simulink model "new_inkine_2020"  (R2022b)
settings: Solver=FixedStepAuto  StartTime=0.0  StopTime=250  FixedStep=0.001  RelTol=1e-3
PreLoadFcn:
  | parameters_new;
InitFcn:
  | parameters_new;
(part 2 of 3)

== matlab function new_inkine_2020/MATLAB Function12 ==
  data: t input; dpt output; V output; a output; flag input
function [dpt,V,a] =TRACE_Pose_experiment(t,flag)%轨迹规划
  % 定义各点坐标
    P1 = [0, 200, 1150];
    P2 = [-160, 40, 1030];
    P3 = [160, 40, 1030];
    P4 = [160, 360, 1270];
    P5 = [-160, 360, 1270];
    % 假设每个阶段运动时间为 x 秒，总运动时间为 xx 秒
     % 计算各段路径的位移
    disp_P1_P5 = norm(P5 - P1);
    disp_P5_P4 = norm(P4 - P5);
    disp_P4_P3 = norm(P3 - P4);
    disp_P3_P2 = norm(P2 - P3);
    disp_P2_P1 = norm(P1 - P2);

    % 第一段运动时间不少于 5 秒
    t1 = 10;

    % 计算速度
    v = disp_P1_P5 / t1;

    % 计算其他段的运动时间
    t2 = disp_P5_P4 / v;
    t3 = disp_P4_P3 / v;
    t4 = disp_P3_P2 / v;
    t5 = disp_P2_P1 / v;

    % 总运动时间
    total_time = t1 + t2 + t3 + t4 + t5;
    if flag == 0
     % P1 -> P5
        [K_1, KV_1, Ka_1] = polynomial_v(t, t1, P1(1), 0, 0, P5(1), 0, 0);
        [S_1, SV_1, Sa_1] = polynomial_v(t, t1, P1(2), 0, 0, P5(2), 0, 0);
        [Z_1, ZV_1, Za_1] = polynomial_v(t, t1, P1(3), 0, 0, P5(3), 0, 0);
        % P5 -> P4
        [K_2, KV_2, Ka_2] = polynomial_v((t - t1), t2, P5(1), 0, 0, P4(1), 0, 0);
        [S_2, SV_2, Sa_2] = polynomial_v((t - t1), t2, P5(2), 0, 0, P4(2), 0, 0);
        [Z_2, ZV_2, Za_2] = polynomial_v((t - t1), t2, P5(3), 0, 0, P4(3), 0, 0);
        % P4 -> P3
        [K_3, KV_3, Ka_3] = polynomial_v((t - t1 - t2), t3, P4(1), 0, 0, P3(1), 0, 0);
        [S_3, SV_3, Sa_3] = polynomial_v((t - t1 - t2), t3, P4(2), 0, 0, P3(2), 0, 0);
        [Z_3, ZV_3, Za_3] = polynomial_v((t - t1 - t2), t3, P4(3), 0, 0, P3(3), 0, 0);
        % P3 -> P2
        [K_4, KV_4, Ka_4] = polynomial_v((t - t1 - t2 - t3), t4, P3(1), 0, 0, P2(1), 0, 0);
        [S_4, SV_4, Sa_4] = polynomial_v((t - t1 - t2 - t3), t4, P3(2), 0, 0, P2(2), 0, 0);
        [Z_4, ZV_4, Za_4] = polynomial_v((t - t1 - t2 - t3), t4, P3(3), 0, 0, P2(3), 0, 0);
        % P2 -> P1
        [K_5, KV_5, Ka_5] = polynomial_v((t - t1 - t2 - t3 - t4), t5, P2(1), 0, 0, P1(1), 0, 0);
        [S_5, SV_5, Sa_5] = polynomial_v((t - t1 - t2 - t3 - t4), t5, P2(2), 0, 0, P1(2), 0, 0);
        [Z_5, ZV_5, Za_5] = polynomial_v((t - t1 - t2 - t3 - t4), t5, P2(3), 0, 0, P1(3), 0, 0);

        % 组合各个阶段的位置
        X = K_1.*(t >= 0 & t < t1) + K_2.*(t >= t1 & t < t1 + t2) + K_3.*(t >= t1 + t2 & t < t1 + t2 + t3) + K_4.*(t >= t1 + t2 + t3 & t < t1 + t2 + t3 + t4) + K_5.*(t >= t1 + t2 + t3 + t4 & t <= total_time);
        Y = S_1.*(t >= 0 & t < t1) + S_2.*(t >= t1 & t < t1 + t2) + S_3.*(t >= t1 + t2 & t < t1 + t2 + t3) + S_4.*(t >= t1 + t2 + t3 & t < t1 + t2 + t3 + t4) + S_5.*(t >= t1 + t2 + t3 + t4 & t <= total_time);
        Z = Z_1.*(t >= 0 & t < t1) + Z_2.*(t >= t1 & t < t1 + t2) + Z_3.*(t >= t1 + t2 & t < t1 + t2 + t3) + Z_4.*(t >= t1 + t2 + t3 & t < t1 + t2 + t3 + t4) + Z_5.*(t >= t1 + t2 + t3 + t4 & t <= total_time);

        % 组合各个阶段的速度
        VX = KV_1.*(t >= 0 & t < t1) + KV_2.*(t >= t1 & t < t1 + t2) + KV_3.*(t >= t1 + t2 & t < t1 + t2 + t3) + KV_4.*(t >= t1 + t2 + t3 & t < t1 + t2 + t3 + t4) + KV_5.*(t >= t1 + t2 + t3 + t4 & t <= total_time);
        VY = SV_1.*(t >= 0 & t < t1) + SV_2.*(t >= t1 & t < t1 + t2) + SV_3.*(t >= t1 + t2 & t < t1 + t2 + t3) + SV_4.*(t >= t1 + t2 + t3 & t < t1 + t2 + t3 + t4) + SV_5.*(t >= t1 + t2 + t3 + t4 & t <= total_time);
        VZ = ZV_1.*(t >= 0 & t < t1) + ZV_2.*(t >= t1 & t < t1 + t2) + ZV_3.*(t >= t1 + t2 & t < t1 + t2 + t3) + ZV_4.*(t >= t1 + t2 + t3 & t < t1 + t2 + t3 + t4) + ZV_5.*(t >= t1 + t2 + t3 + t4 & t <= total_time);

        % 组合各个阶段的加速度
        aX = Ka_1.*(t >= 0 & t < t1) + Ka_2.*(t >= t1 & t < t1 + t2) + Ka_3.*(t >= t1 + t2 & t < t1 + t2 + t3) + Ka_4.*(t >= t1 + t2 + t3 & t < t1 + t2 + t3 + t4) + Ka_5.*(t >= t1 + t2 + t3 + t4 & t <= total_time);
        aY = Sa_1.*(t >= 0 & t < t1) + Sa_2.*(t >= t1 & t < t1 + t2) + Sa_3.*(t >= t1 + t2 & t < t1 + t2 + t3) + Sa_4.*(t >= t1 + t2 + t3 & t < t1 + t2 + t3 + t4) + Sa_5.*(t >= t1 + t2 + t3 + t4 & t <= total_time);
        aZ = Za_1.*(t >= 0 & t < t1) + Za_2.*(t >= t1 & t < t1 + t2) + Za_3.*(t >= t1 + t2 & t < t1 + t2 + t3) + Za_4.*(t >= t1 + t2 + t3 & t < t1 + t2 + t3 + t4) + Za_5.*(t >= t1 + t2 + t3 + t4 & t <= total_time);

        dpt = [X, Y, Z];
        V = [VX, VY, VZ];
        a = [aX, aY, aZ].';

%     elseif flag==1
    else
        [K_1, KV_1, Ka_1] = polynomial_v(t, 2, 0, 0, 0, -150, -100, 0); % 4-6
        [K_2, KV_2, Ka_2] = polynomial_v((t-2), 1, -150, -100, 0, -250, -100, 0); % 6-7
        [K_3, KV_3, Ka_3] = polynomial_v((t-3), 1, -250, -100, 0, -350, -100, 0); % 7-8
        [K_4, KV_4, Ka_4] = polynomial_v((t-4), 2, -350, -100, 0, -500, 0, 0); % 8-10
        K_5 = -500; KV_5 = 0; Ka_5 = 0;
        X = K_1.*(t>=0 & t<2) + K_2.*(t>=2 & t<3) + K_3.*(t>=3 & t<4) + K_4.*(t>=4 & t<6) + K_5.*(t>=6 & t<=10);
        VX = KV_1.*(t>=0 & t<2) + KV_2.*(t>=2 & t<3) + KV_3.*(t>=3 & t<4) + KV_4.*(t>=4 & t<6) + KV_5.*(t>=6 & t<=10);
        aX = Ka_1.*(t>=0 & t<2) + Ka_2.*(t>=2 & t<3) + Ka_3.*(t>=3 & t<4) + Ka_4.*(t>=4 & t<6) + Ka_5.*(t>=6 & t<=10);

        [S_1, SV_1, Sa_1] = polynomial_v(t, 2, 500, 0, 0, 420, -96, -12); % 4-6s
        [S_2, SV_2, Sa_2] = polynomial_v((t-2), 1, 420, -96, -12, 330, -82, 17); % 6-7s
        [S_3, SV_3, Sa_3] = polynomial_v((t-3), 1, 330, -82, 17, 255, -69, 23); % 7-8s
        [S_4, SV_4, Sa_4] = polynomial_v((t-4), 2, 255, -69, 23, 200, 0, 0); % 8-10s
        S_5 = 200; SV_5 = 0; Sa_5 = 0;
        Y = S_1.*(t>=0 & t<2) + S_2.*(t>=2 & t<3) + S_3.*(t>=3 & t<4) + S_4.*(t>=4 & t<6) + S_5.*(t>=6 & t<=10);
        VY = SV_1.*(t>=0 & t<2) + SV_2.*(t>=2 & t<3) + SV_3.*(t>=3 & t<4) + SV_4.*(t>=4 & t<6) + SV_5.*(t>=6 & t<=10);
        aY = Sa_1.*(t>=0 & t<2) + Sa_2.*(t>=2 & t<3) + Sa_3.*(t>=3 & t<4) + Sa_4.*(t>=4 & t<6) + Sa_5.*(t>=6 & t<=10);

        [Z_1, ZV_1, Za_1] = polynomial_v((t-6), 4, 950, 0, 0, 1200, 0, 0);
        Z_2 = 950; ZV_2 = 0; Za_2 = 0;
        Z = Z_2.*(t>=0 & t<6) + Z_1.*(t>=6 & t<=10);
        VZ = ZV_2.*(t>=0 & t<6) + ZV_1.*(t>=6 & t<=10);
        aZ = Za_2.*(t>=0 & t<6) + Za_1.*(t>=6 & t<=10);

        dpt=[X,Y,Z];V=[VX,VY,VZ]; a=[aX,aY,aZ].';

    end
end

== matlab function new_inkine_2020/MATLAB Function13 ==
  data: t input; dpt output; V output; a output; flag input
function [dpt,V,a] =TRACE_Pose_experiment(t,flag)%轨迹规划
  % 定义各点坐标
    P1 = [0, 200, 1150];
    P2 = [-160, 40, 1030];
    P3 = [160, 40, 1030];
    P4 = [160, 360, 1270];
    P5 = [-160, 360, 1270];
    
    % 计算各段路径的位移
    disp_P1_P5 = norm(P5 - P1);
    disp_P5_P4 = norm(P4 - P5);
    disp_P4_P3 = norm(P3 - P4);
    disp_P3_P2 = norm(P2 - P3);
    disp_P2_P1 = norm(P1 - P2);

    % 第一段运动时间不少于 5 秒
    t1 = 10;

    % 计算速度
    v = disp_P1_P5 / t1;

    % 计算其他段的运动时间
    t2 = disp_P5_P4 / v;
    t3 = disp_P4_P3 / v;
    t4 = disp_P3_P2 / v;
    t5 = disp_P2_P1 / v;

    % 单周期总运动时间
    total_time = t1 + t2 + t3 + t4 + t5;
    % 30周期总时间
    total_cycle_time = 30 * total_time;

    if flag == 0
        % 计算时间在30个周期内的相对时间
        t_mod = t - total_time * floor(t / total_time);
        
        % P1 -> P5
        [K_1, KV_1, Ka_1] = polynomial_v(t_mod, t1, P1(1), 0, 0, P5(1), 0, 0);
        [S_1, SV_1, Sa_1] = polynomial_v(t_mod, t1, P1(2), 0, 0, P5(2), 0, 0);
        [Z_1, ZV_1, Za_1] = polynomial_v(t_mod, t1, P1(3), 0, 0, P5(3), 0, 0);
        
        % P5 -> P4
        [K_2, KV_2, Ka_2] = polynomial_v(t_mod - t1, t2, P5(1), 0, 0, P4(1), 0, 0);
        [S_2, SV_2, Sa_2] = polynomial_v(t_mod - t1, t2, P5(2), 0, 0, P4(2), 0, 0);
        [Z_2, ZV_2, Za_2] = polynomial_v(t_mod - t1, t2, P5(3), 0, 0, P4(3), 0, 0);
        
        % P4 -> P3
        [K_3, KV_3, Ka_3] = polynomial_v(t_mod - t1 - t2, t3, P4(1), 0, 0, P3(1), 0, 0);
        [S_3, SV_3, Sa_3] = polynomial_v(t_mod - t1 - t2, t3, P4(2), 0, 0, P3(2), 0, 0);
        [Z_3, ZV_3, Za_3] = polynomial_v(t_mod - t1 - t2, t3, P4(3), 0, 0, P3(3), 0, 0);
        
        % P3 -> P2
        [K_4, KV_4, Ka_4] = polynomial_v(t_mod - t1 - t2 - t3, t4, P3(1), 0, 0, P2(1), 0, 0);
        [S_4, SV_4, Sa_4] = polynomial_v(t_mod - t1 - t2 - t3, t4, P3(2), 0, 0, P2(2), 0, 0);
        [Z_4, ZV_4, Za_4] = polynomial_v(t_mod - t1 - t2 - t3, t4, P3(3), 0, 0, P2(3), 0, 0);
        
        % P2 -> P1
        [K_5, KV_5, Ka_5] = polynomial_v(t_mod - t1 - t2 - t3 - t4, t5, P2(1), 0, 0, P1(1), 0, 0);
        [S_5, SV_5, Sa_5] = polynomial_v(t_mod - t1 - t2 - t3 - t4, t5, P2(2), 0, 0, P1(2), 0, 0);
        [Z_5, ZV_5, Za_5] = polynomial_v(t_mod - t1 - t2 - t3 - t4, t5, P2(3), 0, 0, P1(3), 0, 0);

        % 组合各个阶段的位置（限制在30个周期内）
        X = K_1.*(t_mod >= 0 & t_mod < t1) + ...
            K_2.*(t_mod >= t1 & t_mod < t1 + t2) + ...
            K_3.*(t_mod >= t1 + t2 & t_mod < t1 + t2 + t3) + ...
            K_4.*(t_mod >= t1 + t2 + t3 & t_mod < t1 + t2 + t3 + t4) + ...
            K_5.*(t_mod >= t1 + t2 + t3 + t4 & t_mod <= total_time) .* (t <= total_cycle_time);
        
        Y = S_1.*(t_mod >= 0 & t_mod < t1) + ...
            S_2.*(t_mod >= t1 & t_mod < t1 + t2) + ...
            S_3.*(t_mod >= t1 + t2 & t_mod < t1 + t2 + t3) + ...
            S_4.*(t_mod >= t1 + t2 + t3 & t_mod < t1 + t2 + t3 + t4) + ...
            S_5.*(t_mod >= t1 + t2 + t3 + t4 & t_mod <= total_time) .* (t <= total_cycle_time);
        
        Z = Z_1.*(t_mod >= 0 & t_mod < t1) + ...
            Z_2.*(t_mod >= t1 & t_mod < t1 + t2) + ...
            Z_3.*(t_mod >= t1 + t2 & t_mod < t1 + t2 + t3) + ...
            Z_4.*(t_mod >= t1 + t2 + t3 & t_mod < t1 + t2 + t3 + t4) + ...
            Z_5.*(t_mod >= t1 + t2 + t3 + t4 & t_mod <= total_time) .* (t <= total_cycle_time);

        % 组合各个阶段的速度
        VX = KV_1.*(t_mod >= 0 & t_mod < t1) + ...
             KV_2.*(t_mod >= t1 & t_mod < t1 + t2) + ...
             KV_3.*(t_mod >= t1 + t2 & t_mod < t1 + t2 + t3) + ...
             KV_4.*(t_mod >= t1 + t2 + t3 & t_mod < t1 + t2 + t3 + t4) + ...
             KV_5.*(t_mod >= t1 + t2 + t3 + t4 & t_mod <= total_time) .* (t <= total_cycle_time);
             
        VY = SV_1.*(t_mod >= 0 & t_mod < t1) + ...
             SV_2.*(t_mod >= t1 & t_mod < t1 + t2) + ...
             SV_3.*(t_mod >= t1 + t2 & t_mod < t1 + t2 + t3) + ...
             SV_4.*(t_mod >= t1 + t2 + t3 & t_mod < t1 + t2 + t3 + t4) + ...
             SV_5.*(t_mod >= t1 + t2 + t3 + t4 & t_mod <= total_time) .* (t <= total_cycle_time);
             
        VZ = ZV_1.*(t_mod >= 0 & t_mod < t1) + ...
             ZV_2.*(t_mod >= t1 & t_mod < t1 + t2) + ...
             ZV_3.*(t_mod >= t1 + t2 & t_mod < t1 + t2 + t3) + ...
             ZV_4.*(t_mod >= t1 + t2 + t3 & t_mod < t1 + t2 + t3 + t4) + ...
             ZV_5.*(t_mod >= t1 + t2 + t3 + t4 & t_mod <= total_time) .* (t <= total_cycle_time);

        % 组合各个阶段的加速度
        aX = Ka_1.*(t_mod >= 0 & t_mod < t1) + ...
             Ka_2.*(t_mod >= t1 & t_mod < t1 + t2) + ...
             Ka_3.*(t_mod >= t1 + t2 & t_mod < t1 + t2 + t3) + ...
             Ka_4.*(t_mod >= t1 + t2 + t3 & t_mod < t1 + t2 + t3 + t4) + ...
             Ka_5.*(t_mod >= t1 + t2 + t3 + t4 & t_mod <= total_time) .* (t <= total_cycle_time);
             
        aY = Sa_1.*(t_mod >= 0 & t_mod < t1) + ...
             Sa_2.*(t_mod >= t1 & t_mod < t1 + t2) + ...
             Sa_3.*(t_mod >= t1 + t2 & t_mod < t1 + t2 + t3) + ...
             Sa_4.*(t_mod >= t1 + t2 + t3 & t_mod < t1 + t2 + t3 + t4) + ...
             Sa_5.*(t_mod >= t1 + t2 + t3 + t4 & t_mod <= total_time) .* (t <= total_cycle_time);
             
        aZ = Za_1.*(t_mod >= 0 & t_mod < t1) + ...
             Za_2.*(t_mod >= t1 & t_mod < t1 + t2) + ...
             Za_3.*(t_mod >= t1 + t2 & t_mod < t1 + t2 + t3) + ...
             Za_4.*(t_mod >= t1 + t2 + t3 & t_mod < t1 + t2 + t3 + t4) + ...
             Za_5.*(t_mod >= t1 + t2 + t3 + t4 & t_mod <= total_time) .* (t <= total_cycle_time);

        dpt = [X, Y, Z];
        V = [VX, VY, VZ];
        a = [aX, aY, aZ].';

    else
        % 保持原flag非0的逻辑不变
        [K_1, KV_1, Ka_1] = polynomial_v(t, 2, 0, 0, 0, -150, -100, 0); % 4-6
        [K_2, KV_2, Ka_2] = polynomial_v((t-2), 1, -150, -100, 0, -250, -100, 0); % 6-7
        [K_3, KV_3, Ka_3] = polynomial_v((t-3), 1, -250, -100, 0, -350, -100, 0); % 7-8
        [K_4, KV_4, Ka_4] = polynomial_v((t-4), 2, -350, -100, 0, -500, 0, 0); % 8-10
        K_5 = -500; KV_5 = 0; Ka_5 = 0;
        X = K_1.*(t>=0 & t<2) + K_2.*(t>=2 & t<3) + K_3.*(t>=3 & t<4) + K_4.*(t>=4 & t<6) + K_5.*(t>=6 & t<=10);
        VX = KV_1.*(t>=0 & t<2) + KV_2.*(t>=2 & t<3) + KV_3.*(t>=3 & t<4) + KV_4.*(t>=4 & t<6) + KV_5.*(t>=6 & t<=10);
        aX = Ka_1.*(t>=0 & t<2) + Ka_2.*(t>=2 & t<3) + Ka_3.*(t>=3 & t<4) + Ka_4.*(t>=4 & t<6) + Ka_5.*(t>=6 & t<=10);

        [S_1, SV_1, Sa_1] = polynomial_v(t, 2, 500, 0, 0, 420, -96, -12); % 4-6s
        [S_2, SV_2, Sa_2] = polynomial_v((t-2), 1, 420, -96, -12, 330, -82, 17); % 6-7s
        [S_3, SV_3, Sa_3] = polynomial_v((t-3), 1, 330, -82, 17, 255, -69, 23); % 7-8s
        [S_4, SV_4, Sa_4] = polynomial_v((t-4), 2, 255, -69, 23, 200, 0, 0); % 8-10s
        S_5 = 200; SV_5 = 0; Sa_5 = 0;
        Y = S_1.*(t>=0 & t<2) + S_2.*(t>=2 & t<3) + S_3.*(t>=3 & t<4) + S_4.*(t>=4 & t<6) + S_5.*(t>=6 & t<=10);
        VY = SV_1.*(t>=0 & t<2) + SV_2.*(t>=2 & t<3) + SV_3.*(t>=3 & t<4) + SV_4.*(t>=4 & t<6) + SV_5.*(t>=6 & t<=10);
        aY = Sa_1.*(t>=0 & t<2) + Sa_2.*(t>=2 & t<3) + Sa_3.*(t>=3 & t<4) + Sa_4.*(t>=4 & t<6) + Sa_5.*(t>=6 & t<=10);

        [Z_1, ZV_1, Za_1] = polynomial_v((t-6), 4, 950, 0, 0, 1200, 0, 0);
        Z_2 = 950; ZV_2 = 0; Za_2 = 0;
        Z = Z_2.*(t>=0 & t<6) + Z_1.*(t>=6 & t<=10);
        VZ = ZV_2.*(t>=0 & t<6) + ZV_1.*(t>=6 & t<=10);
        aZ = Za_2.*(t>=0 & t<6) + Za_1.*(t>=6 & t<=10);

        dpt=[X,Y,Z];V=[VX,VY,VZ]; a=[aX,aY,aZ].';

    end
end

== matlab function new_inkine_2020/Velocity ==
  data: dq1 output; dt1 output; dt2 output; dt3 output; q input; v input; dq output
function [dq1,dt1,dt2,dt3,dq] = velocity(q,v)
% L1=2400;L3=2200;S1=557;
x_dot=v(1);y_dot=v(2);z_dot=v(3);
coder.extrinsic('evalin');
L1=0;L3=0;S1=0;R1=0;R2=0;Le=0;K1=0;K2=0;M1=0;M2=0;
L1=evalin('base','L1');L3=evalin('base','L3');S1=evalin('base','S1');R1=evalin('base','R1');Le=evalin('base','Le');R2=evalin('base','R2');
K1=evalin('base','K1');K2=evalin('base','K2');M1=evalin('base','M1');M2=evalin('base','M2');
K2=K1;
theta1=q(1);theta4=q(2);theta5=q(3);
theta7=-pi/6;

% jacobian=[-sin(theta1)*(L1*cos(theta4)+L3*cos(theta5)-S1) -L1*cos(theta1)*sin(theta4) -L3*cos(theta1)*sin(theta5) ;
%     cos(theta1)*(L1*cos(theta4)+L3*cos(theta5)-S1) -L1*sin(theta1)*sin(theta4) -L3*sin(theta1)*sin(theta5) ;
%     0 L1*cos(theta4) L3*cos(theta5) ];
% 
% dq=inv(jacobian)*[x_dot y_dot z_dot].';

inv_jacobian=[-sin(theta1)/(L1*cos(theta1)^2*cos(theta4) - S1*sin(theta1)^2 - S1*cos(theta1)^2 + L3*cos(theta1)^2*cos(theta5) + L1*cos(theta4)*sin(theta1)^2 + L3*cos(theta5)*sin(theta1)^2), cos(theta1)/(L1*cos(theta1)^2*cos(theta4) - S1*sin(theta1)^2 - S1*cos(theta1)^2 + L3*cos(theta1)^2*cos(theta5) + L1*cos(theta4)*sin(theta1)^2 + L3*cos(theta5)*sin(theta1)^2), 0; 
    (cos(theta1)*cos(theta5))/(L1*cos(theta1)^2*cos(theta4)*sin(theta5) - L1*cos(theta1)^2*cos(theta5)*sin(theta4) + L1*cos(theta4)*sin(theta1)^2*sin(theta5) - L1*cos(theta5)*sin(theta1)^2*sin(theta4)), (cos(theta5)*sin(theta1))/(L1*cos(theta1)^2*cos(theta4)*sin(theta5) - L1*cos(theta1)^2*cos(theta5)*sin(theta4) + L1*cos(theta4)*sin(theta1)^2*sin(theta5) - L1*cos(theta5)*sin(theta1)^2*sin(theta4)), sin(theta5)/(L1*cos(theta4)*sin(theta5) - L1*cos(theta5)*sin(theta4)); 
    -(cos(theta1)*cos(theta4))/(L3*cos(theta1)^2*cos(theta4)*sin(theta5) - L3*cos(theta1)^2*cos(theta5)*sin(theta4) + L3*cos(theta4)*sin(theta1)^2*sin(theta5) - L3*cos(theta5)*sin(theta1)^2*sin(theta4)), -(cos(theta4)*sin(theta1))/(L3*cos(theta1)^2*cos(theta4)*sin(theta5) - L3*cos(theta1)^2*cos(theta5)*sin(theta4) + L3*cos(theta4)*sin(theta1)^2*sin(theta5) - L3*cos(theta5)*sin(theta1)^2*sin(theta4)), -sin(theta4)/(L3*cos(theta4)*sin(theta5) - L3*cos(theta5)*sin(theta4))];
dq=inv_jacobian*[x_dot y_dot z_dot].';
dq1=dq(1);
dq4=dq(2);
dq5=dq(3);
theta2=5*pi/6-theta4;theta3=theta7-theta5;
n=sqrt((M1 - R2*cos(theta3))^2 + (M2 - R2*sin(theta3))^2);
J1=-(R1*sin(theta2)+(R1*(K1-R1*sin(theta2))*cos(theta2))/sqrt(Le^2-(K1-R1*sin(theta2))^2));
J2=(R1*cos(theta2)+(R1*(K2-R1*cos(theta2))*sin(theta2))/sqrt(Le^2-(K2-R1*cos(theta2))^2));
J3=(R2*(M2*cos(theta3) - M1*sin(theta3)))/n;
dt1=J1*dq4;
dt2=J2*dq4;
dt3=J3*dq5;
end

== matlab function new_inkine_2020/In_kine ==
  data: q output; theta1 output; t1 output; t2 output; t3 output; dpt input
function [q,theta1,t1,t2,t3]=kine_p(dpt)
% syms S1 S2 L1 L3;

coder.extrinsic('evalin');
L1=0;L3=0;S1=0;S2=0;R1=0;R2=0;Le=0;K1=0;K2=0;M1=0;M2=0;T1=0;T2=0;
L1=evalin('base','L1');L3=evalin('base','L3');S1=evalin('base','S1');S2=evalin('base','S2');R1=evalin('base','R1');Le=evalin('base','Le');R2=evalin('base','R2');
K1=evalin('base','K1');K2=evalin('base','K2');M1=evalin('base','M1');M2=evalin('base','M2');T1=evalin('base','T1');T2=evalin('base','T2');
x=dpt(1);y=dpt(2);z=dpt(3);
if x>0&&y>0
    theta1=atan(y/x);
elseif x>0&&y<0 
    theta1=atan(y/x)+2*pi;
elseif x<0
    theta1=atan(y/x)+pi;
elseif x==0&&y<0 
    theta1=1.5*pi;
elseif x==0&&y>0 
    theta1=0.5*pi;
elseif y==0&&x>0 
    theta1=0;
elseif y==0&&x<0 
    theta1=pi;
else
    theta1=0;
end
%  global theta1;
if x~=0||(x==0&&y==0)
    %大臂转角
    theta4=acos(((z-S2)^2+(x/cos(theta1)+S1)^2+L1^2-L3^2)/(2*L1*((z-S2)^2+(x/cos(theta1)+S1)^2)^0.5))...
    +atan((z-S2)/(x/cos(theta1)+S1));
    %小臂转角
    theta5=-acos(((z-S2)^2+(x/cos(theta1)+S1)^2+L3^2-L1^2)/(2*L3*((z-S2)^2+(x/cos(theta1)+S1)^2)^0.5))...
    +atan((z-S2)/(x/cos(theta1)+S1));
else
    %大臂转角
    theta4=acos(((z-S2)^2+(y/sin(theta1)+S1)^2+L1^2-L3^2)/(2*L1*((z-S2)^2+(y/sin(theta1)+S1)^2)^0.5))...
    +atan((z-S2)/(y/sin(theta1)+S1));
    %小臂转角
    theta5=-acos(((z-S2)^2+(y/sin(theta1)+S1)^2+L3^2-L1^2)/(2*L3*((z-S2)^2+(y/sin(theta1)+S1)^2)^0.5))...
    +atan((z-S2)/(y/sin(theta1)+S1));
end
q=[theta1,theta4,theta5].';
theta2=5*pi/6-theta4;theta3=-pi/6-theta5;
% -X1-T1=t1 三个驱动的位置
t1=-R1*cos(theta2)+(Le^2-(K1-R1*sin(theta2))^2)^0.5-T1;
t2=-R1*sin(theta2)+(Le^2-(K2-R1*cos(theta2))^2)^0.5-T2;
t3=((M1-R2*cos(theta3))^2+(M2-R2*sin(theta3))^2)^0.5;
end
% 
% function [theta1,t1,t2,t3,theta21]=kine_p_2(dpt,delta_q2_all)
% % syms S1 S2 L1 L3;
% X_offest = -25.4;
% Y_offest = 50.520;
% Z_offest = 0.042;
% X_offest = 0;
% Y_offest = 0;
% Z_offest = 0;
% 
% delta_q2 = sum(delta_q2_all, 2);
% % delta_q2 = - delta_q2; 
% K1 = 270; 
% K2 = 270 + delta_q2(17); 
% R1 = 200 + delta_q2(18); 
% R2 = 318 + delta_q2(21); 
% L7 = 414 + delta_q2(19); 
% L8 = 414 + delta_q2(19); 
% M1 = 312.5 + delta_q2(22); 
% M2 = 140.5;
% 
% l_AB = 215 + delta_q2(11);
% l_AD = 600 + delta_q2(5);
% l_CD = 215;
% l_BC = 600 + delta_q2(10);
% l_AE = 150 + delta_q2(13);
% l_DF = 150;
% l_EF = 600 + delta_q2(12);
% l_DK = 550 + delta_q2(7);
% l_DG = 180 + delta_q2(15);
% l_HK = 180;
% l_GH = 550 + delta_q2(14);
% 
% thetaA = pi ;
% thetaB = 5 * pi / 12 ;
% thetaC = 5 * pi / 6 ;
% thetaD = 5 * pi / 6 ;
% 
% a1=80.5037 + delta_q2(3);
% d1=312.5177 + delta_q2(2);
% L2=600 + delta_q2(5);
% L3=550 + delta_q2(7);
% a4=203;
% 
% x=dpt(1);y=dpt(2);z=dpt(3);
% 
% if x<0&&y<0
%     theta1=atan(y/x);
% elseif x<0&&y>0 
%     theta1=atan(y/x)+2*pi;
% elseif x>0
%     theta1=atan(y/x)+pi;
% elseif x==0&&y<0 
%     theta1=0.5*pi;
% elseif x==0&&y>0 
%     theta1=1.5*pi;
% elseif y==0&&x>0 
%     theta1=pi;
% elseif y==0&&x<0 
%     theta1=0;
% else
%     theta1=0;
% end
% %  global theta1;
% if x~=0||(x==0&&y==0)
%     %大臂转角
%     theta2=acos(((z-d1-a4-X_offest)^2+((x-Z_offest*sin(theta1))/cos(theta1)-a1+Y_offest)^2+L2^2-L3^2)/(2*L2*((z-d1-a4-X_offest)^2+((x-Z_offest*sin(theta1))/cos(theta1)-a1+Y_offest)^2)^0.5))...
%     -atan((z-d1-a4-X_offest)/((x-Z_offest*sin(theta1))/cos(theta1)-a1+Y_offest));
%     %小臂转角
%     theta5=acos(((z-d1-a4-X_offest)^2+((x-Z_offest*sin(theta1))/cos(theta1)-a1+Y_offest)^2+L3^2-L2^2)/(2*L3*((z-d1-a4-X_offest)^2+((x-Z_offest*sin(theta1))/cos(theta1)-a1+Y_offest)^2)^0.5))...
%     +atan((z-d1-a4-X_offest)/((x-Z_offest*sin(theta1))/cos(theta1)-a1+Y_offest));
% else
%     %大臂转角
%     theta2=acos(((z-d1-a4-X_offest)^2+((y+Z_offest*cos(theta1))/sin(theta1)-a1+Y_offest)^2+L2^2-L3^2)/(2*L2*((z-d1-a4-X_offest)^2+((y+Z_offest*cos(theta1))/sin(theta1)-a1+Y_offest)^2)^0.5))...
%     -atan((z-d1-a4-X_offest)/((x-Z_offest*sin(theta1))/cos(theta1)-a1+Y_offest));
%     %小臂转角
%     theta5=acos(((z-d1-a4-X_offest)^2+((y+Z_offest*cos(theta1))/sin(theta1)-a1+Y_offest)^2+L3^2-L2^2)/(2*L3*((z-d1-a4-X_offest)^2+((y+Z_offest*cos(theta1))/sin(theta1)-a1+Y_offest)^2)^0.5))...
%     +atan((z-d1-a4-X_offest)/((x-Z_offest*sin(theta1))/cos(theta1)-a1+Y_offest));
% end
% Q1=acos(((z-d1-a4-X_offest)^2+((x-Z_offest*sin(theta1))/cos(theta1)-a1+Y_offest)^2+L3^2-L2^2)/(2*L3*((z-d1-a4-X_offest)^2+((x-Z_offest*sin(theta1))/cos(theta1)-a1+Y_offest)^2)^0.5));
% % Q2=atan(((x-Z_offest*sin(theta1))/cos(theta1)-a1+Y_offest)/(z-d1-a4-X_offest));
% Q3=atan((z-d1-a4-X_offest)/((x-Z_offest*sin(theta1))/cos(theta1)-a1+Y_offest));
% % q=[theta1,theta4,theta5].';
% theta2 = pi - theta2;
% theta5 = pi + theta5;
% theta3=theta5-theta2;
% theta4=2.5*pi-theta5;
% ADC = theta3;
% l_AC = sqrt(l_AD^2 + l_CD^2 - 2*l_AD*l_CD*cos(ADC));
% DAC = acos((l_AD^2 + l_AC^2 - l_CD^2)/(2*l_AD*l_AC));
% BAC = acos((l_AB^2 + l_AC^2 - l_BC^2)/(2*l_AB*l_AC));
% BAD = DAC + BAC;
% theta2_ = 2*pi + theta2 - BAD;
% theta6 = theta2_ - 2*pi + thetaD;
% theta5 = 2*pi - thetaC - theta2;
% t1=R1*cos(theta5)+sqrt(L7^2-(K1-R1*sin(theta5))^2);
% t2=-R1*sin(theta5)+sqrt(L8^2-(K2+R1*cos(theta5))^2);
% t3=sqrt((M1+R2*cos(theta6))^2+(M2+R2*sin(theta6))^2);
% 
% DKH = theta4 - 5*pi/4;
% l_DH = sqrt(l_DK^2 + l_HK^2 - 2*l_DK*l_HK*cos(DKH));
% KDH = acos((l_DK^2 + l_DH^2 - l_HK^2)/(2*l_DK*l_DH));
% GDH = acos((l_DG^2 + l_DH^2 - l_GH^2)/(2*l_DG*l_DH));
% KDG = KDH + GDH;
% FDC = KDG + thetaB - thetaA;
% ADF = theta3 - FDC;
% l_AF = sqrt(l_AD^2 + l_DF^2 - 2*l_AD*l_DF*cos(ADF));
% DAF = acos((l_AD^2 + l_AF^2 - l_DF^2)/(2*l_AD*l_AF));
% EAF = acos((l_AE^2 + l_AF^2 - l_EF^2)/(2*l_AE*l_AF));
% EAD = DAF + EAF;
% theta21 = 2*pi + theta2 - EAD;
% 
% theta1 = theta1 - delta_q2(1);
% t2 = t2 - delta_q2(16);
% t3 = t3 - delta_q2(20);
% end
